simulink subsystem "Odometria"  (R2023b)
settings: Solver=VariableStepAuto  StartTime=0.0  StopTime=10.0  RelTol=1e-3
undefined symbols (not defined in the file): DiscIntNeverNeededParam
settings Model: Creator=ricfe  LastModifiedBy=ricfe

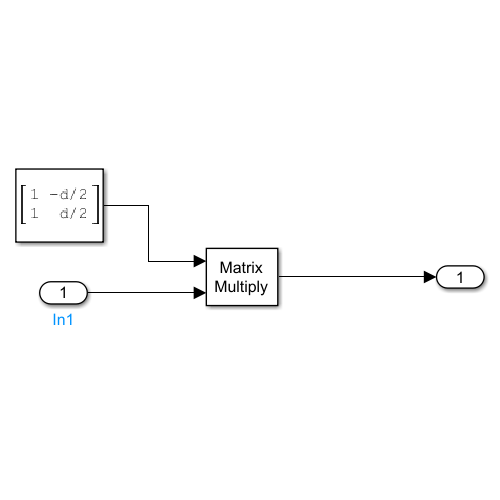
[thumbnail: Simulink's stored preview of the top-level diagram]
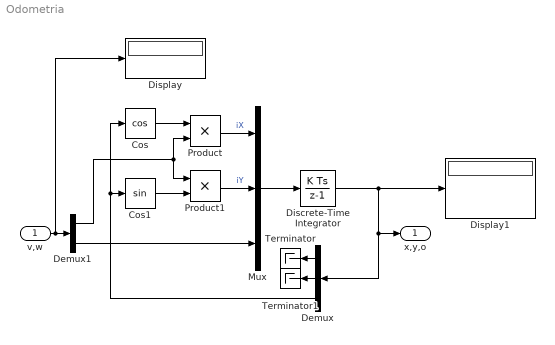
== system Odometria ==
  v,w : Inport
  Cos : Trigonometry  Operator=cos
  Cos1 : Trigonometry
  Demux : Demux  Outputs=3
  Demux1 : Demux  Outputs=2
  Discrete-Time Integrator : DiscreteIntegrator  SampleTime=-1  ICPrevOutput=DiscIntNeverNeededParam  ICPrevScaledInput=DiscIntNeverNeededParam
  Display : Display
  Display1 : Display
  Mux : Mux  Inputs=3
  Product : Product
  Product1 : Product
  Terminator : Terminator
  Terminator1 : Terminator
  x,y,o : Outport
  wires:
  Discrete-Time Integrator/1 -> x,y,o/1, Demux/1, Display1/1
  v,w/1 -> Demux1/1, Display/1
  Demux/1 -> Terminator/1
  Demux/2 -> Terminator1/1
  Demux/3 -> Cos1/1, Cos/1
  Demux1/1 -> Product/2, Product1/1
  Cos1/1 -> Product1/2
  Cos/1 -> Product/1
  Product/1 -> Mux/1  "iX"
  Product1/1 -> Mux/2  "iY"
  Demux1/2 -> Mux/3
  Mux/1 -> Discrete-Time Integrator/1
